simulink model "Project1_Trial"  (R2019a)
settings: Solver=VariableStepAuto  StartTime=0.0  StopTime=10.0  RelTol=1e-3
values from neighbouring files (symbols this model uses):
  X = input(y)    [Project_Trial1_run.m]
settings Model: Creator=razue  LastModifiedBy=razue

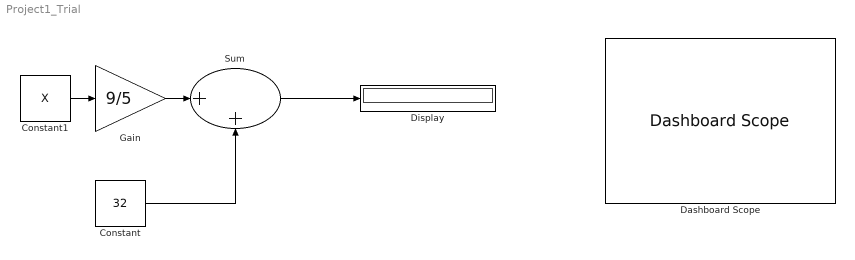
== system Project1_Trial ==
  Constant : Constant  Value=32
  Constant1 : Constant  Value=X  VectorParams1D=off
  Dashboard Scope : DashboardScope
  Display : Display
  Gain : Gain  Gain=9/5
  Sum : Sum  Inputs=|++
  wires:
  Gain/1 -> Sum/1
  Constant/1 -> Sum/2
  Sum/1 -> Display/1
  Constant1/1 -> Gain/1
